simulink model "P1_pt1_2_Variable"  (R2023b)
settings: Solver=VariableStepAuto  StartTime=0.0  StopTime=25  FixedStep=0.001  RelTol=1e-3
undefined symbols (not defined in the file or in its folder): A, b, freq, J, w_0
settings Model: Creator=oscar  LastModifiedBy=oscar

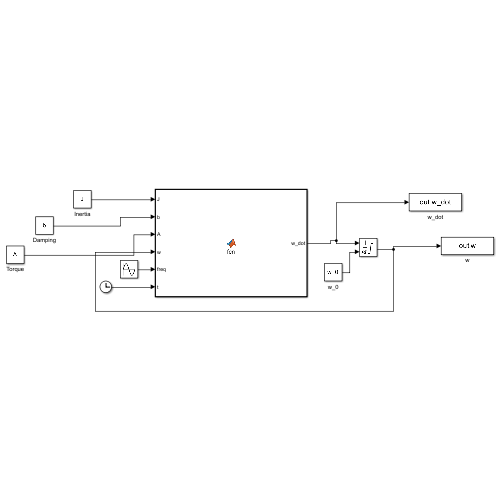
[thumbnail: Simulink's stored preview of the top-level diagram]
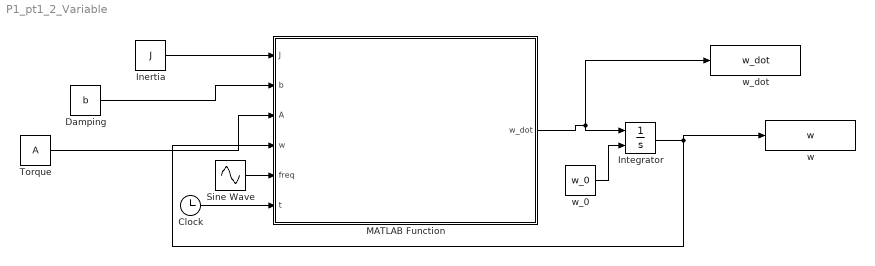
== system P1_pt1_2_Variable ==
  Clock : Clock
  Damping : Constant  Value=b
  Inertia : Constant  Value=J
  Integrator : Integrator  InitialConditionSource=external  LimitOutput=on  UpperSaturationLimit=1000
  MATLAB Function : MATLAB Function  TreatAsAtomicUnit=on
  Sine Wave : Sin  Amplitude=A  Frequency=freq  SampleTime=0
  Torque : Constant  Value=A
  w : ToWorkspace  VariableName=w  SaveFormat=Structure With Time  SampleTime=-1
  w_0 : Constant  Value=w_0
  w_dot : ToWorkspace  VariableName=w_dot  SaveFormat=Structure With Time  SampleTime=-1
  wires:
  MATLAB Function/1(w_dot) -> w_dot/1, Integrator/1
  Inertia/1 -> MATLAB Function/1(J)
  Damping/1 -> MATLAB Function/2(b)
  Torque/1 -> MATLAB Function/3(A)
  Integrator/1 -> w/1, MATLAB Function/4(w)
  w_0/1 -> Integrator/2
  Clock/1 -> MATLAB Function/6(t)
  Sine Wave/1 -> MATLAB Function/5(freq)

== matlab function P1_pt1_2_Variable/MATLAB Function ==
  data: J input; w_dot output; b input; A input; w input; freq input; t input
function w_dot = fcn(J, b, A, w, freq, t)

tau_damped = b*w;
tau = A*sin(freq*t);

w_dot = (1/J)*(A-(b*w));

end
